simulink model "PC_host_SCI_interface_PI"  (R2018b)
settings: Solver=FixedStepDiscrete  StartTime=0.0  StopTime=Inf  RelTol=1e-3  EnableMultiTasking=on
undefined symbols (not defined in the file or in its folder): serial
libraries: instrumentlib x3, simulink x1
settings Model: EnablePacing=on  ExtModeTrigDuration=8  Creator=mocan  LastModifiedBy=mocan
settings OptimizationCC: DefaultUnderspecifiedDataType=single  EnhancedBackFolding=on  PassReuseOutputArgsAs=Individual arguments  MaxStackSize=512  OptimizeBlockOrder=speed  DifferentSizesBufferReuse=on  OptimizationCustomize=off
settings DebuggingCC: ParameterTunabilityLossMsg=error
settings HardwareCC: ProdBitPerChar=16  ProdBitPerInt=16  ProdBitPerPointer=32  ProdBitPerSizeT=32  ProdBitPerPtrDiffT=32  ProdLargestAtomicInteger=Integer  ProdLargestAtomicFloat=None  ProdWordSize=16  ProdLongLongMode=on  ProdHWDeviceType=Texas Instruments->C2000
settings SFSimCC: MATLABDynamicMemAlloc=off
settings RTWCC: SystemTargetFile=ert.tlc  HardwareBoard=TI Delfino F28379D LaunchPad  TemplateMakefile=ert_default_tmf  GenerateReport=on  Toolchain=Texas Instruments Code Composer Studio (C2000)  IncludeHyperlinkInReport=on  LaunchReport=on  GenerateTraceInfo=on  GenerateTraceReport=on  GenerateTraceReportSl=on  GenerateTraceReportSf=on  GenerateTraceReportEml=on
settings CodeAppCC: ForceParamTrailComments=on  IgnoreCustomStorageClasses=off  OperatorAnnotations=on  SimulinkDataObjDesc=on  SFDataObjDesc=on  InsertBlockDesc=on
settings ERTTargetCC: CodeReplacementLibrary=TI C28x  SupportContinuousTime=on

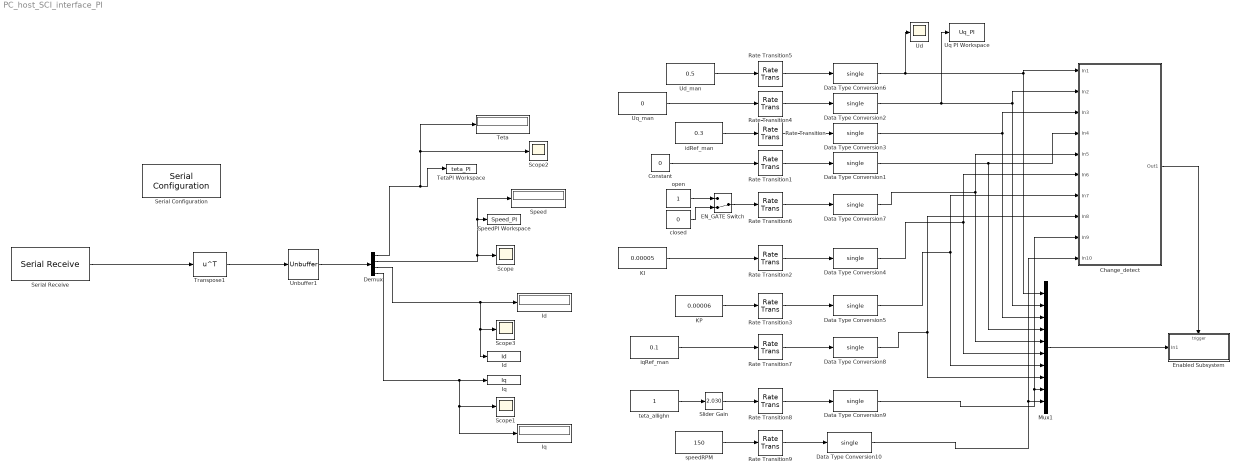
== system PC_host_SCI_interface_PI ==
  Change_detect : Subsystem
  Constant : Constant  Value=0
  Data Type Conversion{1..10} (10 alike) : DataTypeConversion  OutDataTypeStr=single
  Demux : Demux
  EN_GATE Switch : ManualSwitch  CurrentSetting=0
  Enabled Subsystem : Subsystem  TreatAsAtomicUnit=on
  Id : Display
  "Id " : ToWorkspace  VariableName=Id  SaveFormat=Timeseries  SampleTime=-1
  Iq : Display
  "Iq " : ToWorkspace  VariableName=Iq  SaveFormat=Timeseries  SampleTime=-1
  KI : Constant  Value=0.00005
  KP : Constant  Value=0.00006
  Mux1 : Mux  Inputs=10
  Rate Transition{,1..9} (10 alike) : RateTransition
  Scope{,1..3} (4 alike) : Scope
  Serial Configuration : instrumentlib/Serial Configuration  Priority=-200000  ComPortMenu=COM11  ComPort=COM11  ObjConstructor=serial('COM11');  BaudRate=5e6  DataBits=8  Parity=none  StopBits=1  FlowControl=none  Timeout=10  ByteOrder=LittleEndian
  Serial Receive : instrumentlib/Serial Receive  ComPortMenu=COM11  ComPort=COM11  ObjConstructor=serial('COM11');  Header=S  Terminator=E  DataSize="[4  1]"  DataType=single  EnableBlockingMode=on  ActionDataUnavailable=Output last received value  CustomValue=0  SampleTime=0.01
  Slider Gain : simulink/Math Operations/Slider Gain  gain=2.030  low=0  high=7
  "Speed " : Display
  SpeedPI Workspace : ToWorkspace  VariableName=Speed_PI  SaveFormat=Timeseries  SampleTime=-1
  Teta : Display
  TetaPI Workspace : ToWorkspace  VariableName=teta_PI  SaveFormat=Timeseries  SampleTime=-1
  Transpose1 : Math  Operator=transpose  SaturateOnIntegerOverflow=on
  Ud : Scope
  "Ud_man " : Constant  Value=0.5
  Unbuffer1 : Unbuffer
  Uq PI Workspace : ToWorkspace  VariableName=Uq_PI  SaveFormat=Timeseries  SampleTime=-1
  Uq_man : Constant  Value=0
  "closed " : Constant  Value=0
  "idRef_man " : Constant  Value=0.3
  iqRef_man : Constant  Value=0.1
  open : Constant
  speedRPM : Constant  Value=150
  teta_allighn : Constant
  wires:
  Demux/1 -> Scope2/1, Teta/1, TetaPI Workspace/1
  Demux/2 -> "Speed "/1, SpeedPI Workspace/1, Scope/1
  Constant/1 -> Rate Transition1/1
  Rate Transition4/1 -> Data Type Conversion2/1
  Rate Transition/1 -> Data Type Conversion3/1
  Rate Transition1/1 -> Data Type Conversion1/1
  Rate Transition2/1 -> Data Type Conversion4/1
  Rate Transition3/1 -> Data Type Conversion5/1
  Uq_man/1 -> Rate Transition4/1
  "idRef_man "/1 -> Rate Transition/1
  KI/1 -> Rate Transition2/1
  KP/1 -> Rate Transition3/1
  "Ud_man "/1 -> Rate Transition5/1
  Rate Transition5/1 -> Data Type Conversion6/1
  Data Type Conversion2/1 -> Uq PI Workspace/1, Mux1/2, Change_detect/2(In2)
  Data Type Conversion3/1 -> Mux1/3, Change_detect/3(In3)
  Data Type Conversion1/1 -> Mux1/4, Change_detect/4(In4)
  Data Type Conversion4/1 -> Change_detect/6(In6), Mux1/6
  Data Type Conversion5/1 -> Change_detect/7(In7), Mux1/7
  Transpose1/1 -> Unbuffer1/1
  Unbuffer1/1 -> Demux/1
  Mux1/1 -> Enabled Subsystem/1(In1)
  Change_detect/1(Out1) -> Enabled Subsystem/Trigger
  Data Type Conversion6/1 -> Ud/1, Mux1/1, Change_detect/1(In1)
  "closed "/1 -> EN_GATE Switch/2
  Rate Transition6/1 -> Data Type Conversion7/1
  EN_GATE Switch/1 -> Rate Transition6/1
  open/1 -> EN_GATE Switch/1
  Data Type Conversion7/1 -> Change_detect/5("In5 "), Mux1/5
  Demux/3 -> Id/1, Scope3/1, "Id "/1
  Demux/4 -> Scope1/1, Iq/1, "Iq "/1
  Serial Receive/1 -> Transpose1/1
  Data Type Conversion8/1 -> Change_detect/8(In8), Mux1/8
  iqRef_man/1 -> Rate Transition7/1
  Rate Transition7/1 -> Data Type Conversion8/1
  Slider Gain/1 -> Rate Transition8/1
  Rate Transition8/1 -> Data Type Conversion9/1
  Data Type Conversion9/1 -> Change_detect/9(In9), Mux1/9
  teta_allighn/1 -> Slider Gain/1
  Data Type Conversion10/1 -> Change_detect/10(In10), Mux1/10
  Rate Transition9/1 -> Data Type Conversion10/1
  speedRPM/1 -> Rate Transition9/1

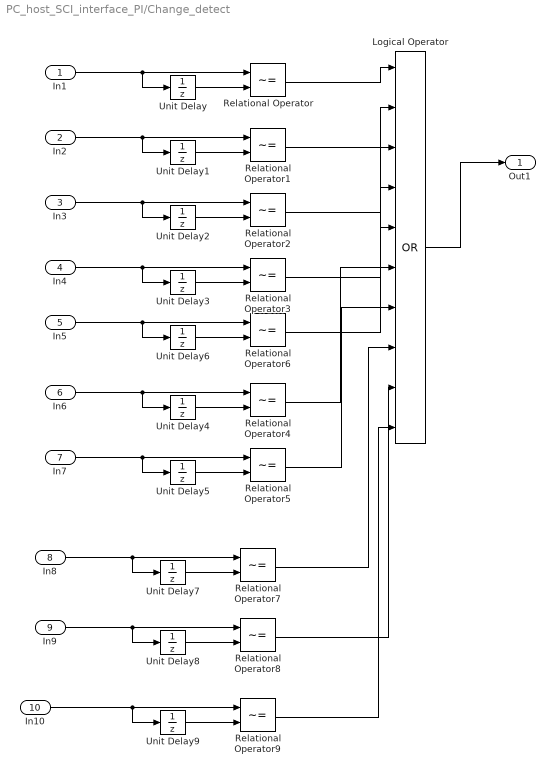
== system PC_host_SCI_interface_PI/Change_detect ==
  In1 : Inport
  In2 : Inport  Port=2
  In3 : Inport  Port=3
  In4 : Inport  Port=4
  "In5 " : Inport  Port=5
  In6 : Inport  Port=6
  In7 : Inport  Port=7
  In8 : Inport  Port=8
  In9 : Inport  Port=9
  In10 : Inport  Port=10
  Logical Operator : Logic  Operator=OR  Inputs=10  AllPortsSameDT=off  OutDataTypeStr=boolean
  Relational Operator{,1..9} (10 alike) : RelationalOperator  Operator=~=  OutDataTypeStr=boolean  RndMeth=Nearest
  Unit Delay{,1..9} (10 alike) : UnitDelay  InitialCondition=0.5  SampleTime=-1
  Out1 : Outport
  wires:
  Unit Delay/1 -> Relational Operator/2
  In1/1 -> Unit Delay/1, Relational Operator/1
  Logical Operator/1 -> Out1/1
  Relational Operator/1 -> Logical Operator/1
  In2/1 -> Relational Operator1/1, Unit Delay1/1
  Unit Delay1/1 -> Relational Operator1/2
  Relational Operator1/1 -> Logical Operator/2
  Relational Operator2/1 -> Logical Operator/3
  Unit Delay2/1 -> Relational Operator2/2
  In3/1 -> Unit Delay2/1, Relational Operator2/1
  In4/1 -> Relational Operator3/1, Unit Delay3/1
  Unit Delay3/1 -> Relational Operator3/2
  Relational Operator3/1 -> Logical Operator/4
  Unit Delay4/1 -> Relational Operator4/2
  In6/1 -> Unit Delay4/1, Relational Operator4/1
  In7/1 -> Relational Operator5/1, Unit Delay5/1
  Unit Delay5/1 -> Relational Operator5/2
  Relational Operator5/1 -> Logical Operator/7
  Relational Operator4/1 -> Logical Operator/6
  Relational Operator6/1 -> Logical Operator/5
  Unit Delay6/1 -> Relational Operator6/2
  "In5 "/1 -> Unit Delay6/1, Relational Operator6/1
  Relational Operator7/1 -> Logical Operator/8
  Unit Delay7/1 -> Relational Operator7/2
  In8/1 -> Unit Delay7/1, Relational Operator7/1
  Relational Operator8/1 -> Logical Operator/9
  In9/1 -> Relational Operator8/1, Unit Delay8/1
  Unit Delay8/1 -> Relational Operator8/2
  Unit Delay9/1 -> Relational Operator9/2
  In10/1 -> Unit Delay9/1, Relational Operator9/1
  Relational Operator9/1 -> Logical Operator/10

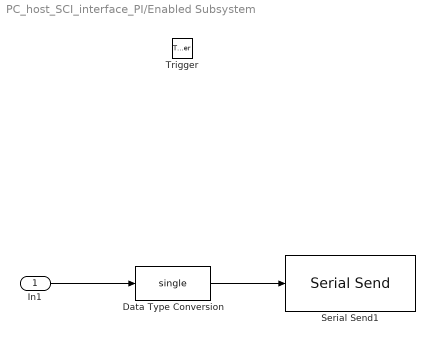
== system PC_host_SCI_interface_PI/Enabled Subsystem ==
  In1 : Inport
  Trigger : TriggerPort  VariantControl=Variant  PortDimensions=1
  Data Type Conversion : DataTypeConversion  OutDataTypeStr=single  ConvertRealWorld=Stored Integer (SI)
  Serial Send1 : instrumentlib/Serial Send  ComPortMenu=COM11  ComPort=COM11  ObjConstructor=serial('COM11');  Header=SS  Terminator=EE  EnableBlockingMode=on
  wires:
  In1/1 -> Data Type Conversion/1
  Data Type Conversion/1 -> Serial Send1/1
